simulink model "hybrid_gwo_pso_mppt_grid_det"  (R2024a)
settings: Solver=FixedStepDiscrete  StartTime=0.0  StopTime=2.5  RelTol=1e-3
PreLoadFcn:
  | Ts_Power=1e-6;
  | Ts_Control=100e-6;
undefined symbols (not defined in the file or in its folder): D1, Delta, sigbuilder_block
libraries: spsSeriesRLCBranchLib x5, spsMeanLib x3, spsThreePhaseTransformerTwoWindingsLib x2, spsDistributedParametersLineLib x2, spsThreePhaseParallelRLCLoadLib x2, slpidlib x2, spsabctodq0Lib x2, spsVoltageMeasurementLib x2, spsPWMGeneratorDCDCLib x1, spsThreePhaseSeriesRLCLoadLib x1, spsThreeLevelBridgeLib x1, spsThreePhaseSourceLib x1
(part 2 of 2)

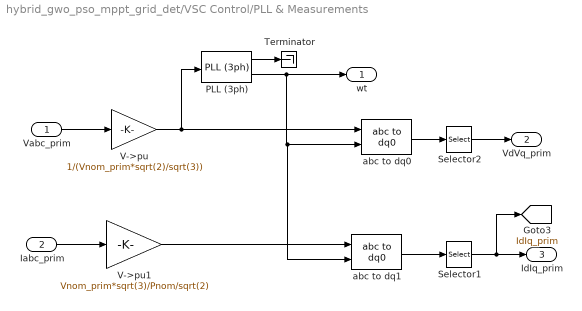
== system hybrid_gwo_pso_mppt_grid_det/VSC Control/PLL & Measurements ==
  Vabc_prim : Inport
  Iabc_prim : Inport  Port=2
  PLL (3ph) : spsPLL3phLib/PLL (3ph)  Fmin=45  Par_Init="[-0.57  Fnom]"  ParK=[180, 3200, 1]  TcD=1e-4  MaxRateChangeFreq=12  FilterCutOffFreq=25  Ts=Ts  AGC=on
  Selector1 : Selector  InputPortWidth=3  IndexOptions=Index vector (dialog)  Indices=[1 2]  OutputSizes=1
  Selector2 : Selector  InputPortWidth=3  IndexOptions=Index vector (dialog)  Indices=[1 2]  OutputSizes=1
  Terminator : Terminator
  V->pu : Gain  Gain=1/(Vnom_prim*sqrt(2)/sqrt(3))  SaturateOnIntegerOverflow=on  OutDataTypeStr=Inherit: Same as input  ParamDataTypeStr=Inherit: Same as input
  V->pu1 : Gain  Gain=Vnom_prim*sqrt(3)/Pnom/sqrt(2)  SaturateOnIntegerOverflow=on  OutDataTypeStr=Inherit: Same as input  ParamDataTypeStr=Inherit: Same as input
  abc to dq0 : spsabctodq0Lib/abc to dq0  Alignment=90 degrees behind phase A axis
  abc to dq1 : spsabctodq0Lib/abc to dq0  Alignment=90 degrees behind phase A axis
  wt : Outport  VectorParamsAs1DForOutWhenUnconnected=off
  VdVq_prim : Outport  Port=2  VectorParamsAs1DForOutWhenUnconnected=off
  IdIq_prim : Outport  Port=3  VectorParamsAs1DForOutWhenUnconnected=off
  tag scope: IdIq_prim=global
  wires:
  V->pu1/1 -> abc to dq1/1
  V->pu/1 -> PLL (3ph)/1, abc to dq0/1
  abc to dq1/1 -> Selector1/1
  Vabc_prim/1 -> V->pu/1
  Iabc_prim/1 -> V->pu1/1
  abc to dq0/1 -> Selector2/1
  Selector2/1 -> VdVq_prim/1
  Selector1/1 -> [IdIq_prim], IdIq_prim/1
  PLL (3ph)/2 -> wt/1, abc to dq1/2, abc to dq0/2
  PLL (3ph)/1 -> Terminator/1

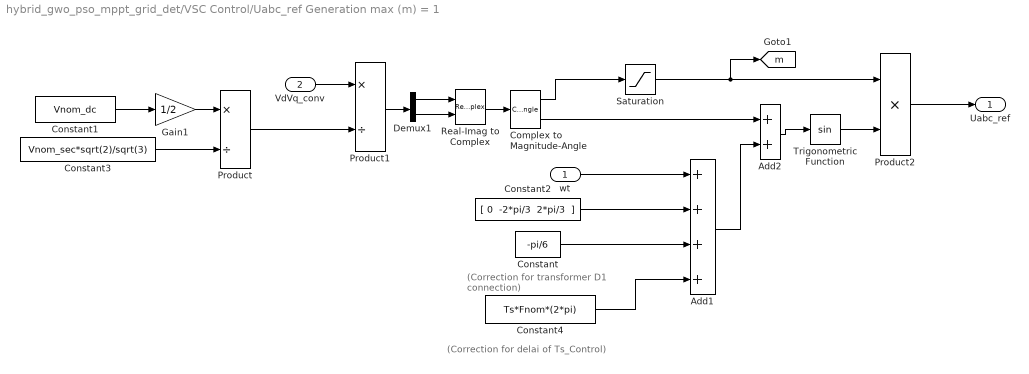
== system hybrid_gwo_pso_mppt_grid_det/VSC Control/Uabc_ref Generation max (m) = 1 ==
  note: (Correction for transformer
      |  D1 connection)
  note: (Correction for delai of Ts_Control)
  wt : Inport
  VdVq_conv : Inport  Port=2
  Add1 : Sum  Inputs=++++
  Add2 : Sum
  Complex to Magnitude-Angle : ComplexToMagnitudeAngle
  Constant : Constant  Value=-pi/6
  Constant1 : Constant  Value=Vnom_dc
  Constant2 : Constant  Value="[ 0  -2*pi/3  2*pi/3  ]"
  Constant3 : Constant  Value=Vnom_sec*sqrt(2)/sqrt(3)
  Constant4 : Constant  Value=Ts*Fnom*(2*pi)
  Demux1 : Demux  Outputs=2
  Gain1 : Gain  Gain=1/2
  Product : Product  Inputs=*/  RndMeth=Zero
  Product1 : Product  Inputs=*/  RndMeth=Zero
  Product2 : Product  Inputs=**  RndMeth=Zero
  Real-Imag to Complex : RealImagToComplex
  Saturation : Saturate  UpperLimit=1  LowerLimit=0
  Trigonometric Function : Trigonometry
  Uabc_ref : Outport  VectorParamsAs1DForOutWhenUnconnected=off
  tag scope: m=global
  wires:
  Complex to Magnitude-Angle/1 -> Saturation/1
  Constant1/1 -> Gain1/1
  VdVq_conv/1 -> Product1/1
  Product1/1 -> Demux1/1
  Gain1/1 -> Product/1
  Real-Imag to Complex/1 -> Complex to Magnitude-Angle/1
  Demux1/1 -> Real-Imag to Complex/1
  Demux1/2 -> Real-Imag to Complex/2
  Constant2/1 -> Add1/2
  Constant/1 -> Add1/3
  Constant3/1 -> Product/2
  Product/1 -> Product1/2
  Complex to Magnitude-Angle/2 -> Add2/1
  Add1/1 -> Add2/2
  Add2/1 -> Trigonometric Function/1
  Saturation/1 -> [m], Product2/1
  Trigonometric Function/1 -> Product2/2
  Product2/1 -> Uabc_ref/1
  wt/1 -> Add1/1
  Constant4/1 -> Add1/4

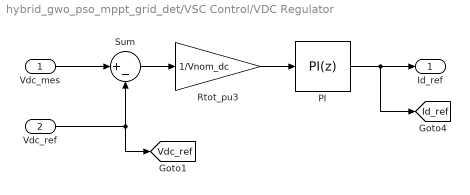
== system hybrid_gwo_pso_mppt_grid_det/VSC Control/VDC Regulator ==
  Vdc_mes : Inport  PortDimensions=1
  Vdc_ref : Inport  Port=2  PortDimensions=1
  PI : slpidlib/PID Controller  Controller=PI  Form=Parallel  TimeDomain=Discrete-time  UseExternalTs=off  SampleTime=Ts  IntegratorMethod=Trapezoidal  FilterMethod=Forward Euler  ControllerParametersSource=internal  P=Kp_VDCreg  I=Ki_VDCreg  UseKiTs=off  D=0  UseExternalDerivativeSource=off  N=100  UseFilter=on  TunerSelectOption=Transfer Function Based (PID Tuner App)  InitialConditionSource=internal  InitialConditionForIntegrator=0  InitialConditionForFilter=0  DifferentiatorICPrevScaledInput=0  ExternalReset=none  TrackingMode=off  Kt=1  LimitOutput=on  SatLimitsSource=internal  UpperSaturationLimit=1.5  LowerSaturationLimit=-1.5  LinearizeAsGain=off  AntiWindupMode=none  Kb=1  LimitIntegrator=off  UpperIntegratorSaturationLimit=inf  LowerIntegratorSaturationLimit=-inf  POutMin=[]  POutMax=[]  IOutMin=[]  IOutMax=[]  DOutMin=[]  DOutMax=[]  NOutMin=[]  NOutMax=[]  SumOutMin=[]  SumOutMax=[]  SaturationOutMin=[]  SaturationOutMax=[]  PParamMin=[]  PParamMax=[]  IParamMin=[]  IParamMax=[]  DParamMin=[]  DParamMax=[]  NParamMin=[]  NParamMax=[]  KbParamMin=[]  KbParamMax=[]  KtParamMin=[]  KtParamMax=[]  KbOutMin=[]  KbOutMax=[]  KtOutMin=[]  KtOutMax=[]  IntegratorOutMin=[]  IntegratorOutMax=[]  FilterOutMin=[]  FilterOutMax=[]  SumI1OutMin=[]  SumI1OutMax=[]  SumI2OutMin=[]  SumI2OutMax=[]  SumI3OutMin=[]  SumI3OutMax=[]  SumI4OutMin=[]  SumI4OutMax=[]  SumDOutMin=[]  SumDOutMax=[]  DifferentiatorOutMin=[]  DifferentiatorOutMax=[]  FilterDiffOutCoefMin=[]  FilterDiffOutCoefMax=[]  ReciprocalOutMin=[]  ReciprocalOutMax=[]  SumDenOutMin=[]  SumDenOutMax=[]  SumNumOutMin=[]  SumNumOutMax=[]  DivideOutMin=[]  DivideOutMax=[]  UdiffTsProdOutMin=[]  UdiffTsProdOutMax=[]  NTsProdOutMin=[]  NTsProdOutMax=[]  UintegralTsProdOutMin=[]  UintegralTsProdOutMax=[]  UngainTsProdOutMin=[]  UngainTsProdOutMax=[]  ClampingZeroOutDataTypeStr=Inherit: Inherit via back propagation  ClampingZeroOutMin=[]  ClampingZeroOutMax=[]  FilterDenConstantOutDataTypeStr=Inherit: Inherit via back propagation  FilterDenConstantOutMin=[]  FilterDenConstantOutMax=[]  PCopyOutDataTypeStr=Inherit: Inherit via back propagation  PCopyOutMin=[]  PCopyOutMax=[]  NCopyOutDataTypeStr=Inherit: Inherit via back propagation  NCopyOutMin=[]  NCopyOutMax=[]  IntegratorContinuousStateAttributes=''  IntegratorStateMustResolveToSignalObject=off  IntegratorRTWStateStorageClass=Auto  FilterContinuousStateAttributes=''  FilterStateMustResolveToSignalObject=off  FilterRTWStateStorageClass=Auto  ParallelPVariant=InternalParameters  IdealPVariant=Disabled  IVariant=InternalParameters  DVariant=Disabled  IntegratorVariant=Discrete  SatVariant=Enabled  AWVariant=Passthrough  PCopyVariant=Disabled  TRVariant=Disabled  FdbkBlocksVariant=Forward  IdealPFdbkVariant=Disabled  SatFdbkVariant=Disabled  DerivativeFilterVariant=Disabled  NVariant=Disabled  NCopyVariant=Disabled_SignalSpec  FilterICVariant=Disabled  IntegratorICVariant=InternalICs  ExternalResetVariant=Disabled  TRSumVariant=Passthrough  SumFdbkVariant=Disabled  SumVariant=Sum_PI  TsampFilterVariant=InternalTs  TsampNgainVariant=Passthrough  TsampIntegralVariant=Disabled_SignalSpec  ExternalSaturationOutDataTypeStr=Inherit: Same as second input  DerivativeSourceVariant=Disabled
  Rtot_pu3 : Gain  Gain=1/Vnom_dc  SaturateOnIntegerOverflow=on  OutDataTypeStr=Inherit: Same as input  ParamDataTypeStr=Inherit: Same as input
  Sum : Sum  Inputs=|+-
  Id_ref : Outport  SampleTime=Ts  InitialOutput=0  VectorParamsAs1DForOutWhenUnconnected=off
  tag scope: Id_ref=global, Vdc_ref=global
  wires:
  Sum/1 -> Rtot_pu3/1
  Vdc_mes/1 -> Sum/1
  Vdc_ref/1 -> Sum/2, [Vdc_ref]
  Rtot_pu3/1 -> PI/1
  PI/1 -> [Id_ref], Id_ref/1

== matlab function hybrid_gwo_pso_mppt_grid_det/ MPPT Controller using GWOPSO /MPPT/MPPT Controller using GWOPSO  ==
  settings: updateMethod=DISCRETE  sampleTime=Ts_Control
  data: Vpv input; Ipv input; Enabled input; D output
%%
% * Author:  Eng. Salah Abbas Taha (S.A.Taha)(salahabbas041@gmail,com,07748191514,Tele.@Eng_441)
% * Date: 06.11.2024
function D = Hybrid_GWO_PSO(Vpv, Ipv,Enabled)
Dinit = 0.5;
SearchAgents_no=6;   % Number of search agents
Max_iteration=10;    % Maximum numbef of iterations
lb = 0.3;            % lb is the lower bound: lb=[lb_1,lb_2,...,lb_d]
ub = 0.9;            % up is the uppper bound: ub=[ub_1,ub_2,...,ub_d]
w=0.5;
a=2;
power_delta =0.01;


% initialize alpha, beta, and delta_pos
persistent params;

if isempty(params)
    params = initialize(SearchAgents_no,lb,ub); 
end



    
% Calculate power
fitness = Vpv * Ipv; 

% Weather conditions test 
if params.runing==false
    
    if abs(fitness - params.power_last) / params.power_last >= power_delta
        params = initialize(SearchAgents_no,lb,ub); 
    else
        D = params.Alpha_pos;
        params.power_last = fitness;
        return;
    end
        
end

params.power_last = fitness;
params.fitness(params.index) = fitness; % Store fitness for the current wolf

% Output duty cycle for the current wolf
D = params.Positions(params.index);

% Step 2: Check if all wolves have been evaluated
params.index = params.index + 1;



if params.index > SearchAgents_no
    
    % Reset index after evaluating all wolves
    params.index = 1; 
    params.iter = params.iter + 1;
    
    % Update dominant levels (alpha, beta, delta)
    [sorted_fitness, sorted_idx] = sort(params.fitness, 'descend');
    params.Alpha_score = sorted_fitness(1); 
    params.Alpha_pos = params.Positions(sorted_idx(1));
    params.Beta_score = sorted_fitness(2); 
    params.Beta_pos = params.Positions(sorted_idx(2));
    params.Delta_score = sorted_fitness(3); 
    params.Delta_pos = params.Positions(sorted_idx(3));
    
    
   
    
    
    for i=1:size(params.Positions,1)
        
        r1=rand(); % r1 is a random number in [0,1]
        r2=rand(); % r2 is a random number in [0,1]
        r3=rand(); % r3 is a random number in [0,1]
        
        A1=2*a*r1-a; 
        C1=2*r2; 
        D_alpha=abs(C1*params.Alpha_pos-w*params.Positions(i)); 
        X1=params.Alpha_pos-A1*D_alpha; 

  
        A2=2*a*r1-a; 
        C2=2*r2; 
        D_beta=abs(C2*params.Beta_pos-w*params.Positions(i)); 
        X2=params.Beta_pos-A2*D_beta; 

       
        A3=2*a*r1-a; 
        C3=2*r2;
        D_delta=abs(C3*params.Delta_pos-w*params.Positions(i)); 
        X3=params.Delta_pos-A3*D_delta; 

        % velocity updation
        params.velocity(i)=w*(params.velocity(i)+C1*r1*(X1-params.Positions(i))+C2*r2*(X2-params.Positions(i))+C3*r3*(X3-params.Positions(i)));
        % positions update
        newPosition = params.Positions(i)+params.velocity(i);
        
        % Enforce boundaries on duty cycle
        if newPosition > ub
            newPosition = ub;
        elseif newPosition < lb
            newPosition = lb;
        end
        
        params.Positions(i)=newPosition;
                   
    end%end for.
    
    
    % Check termination conditions
    if params.iter >= Max_iteration 
%         fprintf('Converged or Max Iterations Reached\n');
        params.runing = false;
        D = params.Alpha_pos;
    end
 
    
end%end if.

if Enabled==0
    D = Dinit;
end


end%end function.


function params = initialize(SearchAgents_no,lb,ub)

params.Alpha_pos= 0;
params.Alpha_score = 0; 

params.Beta_pos=0;
params.Beta_score=0; 
params.Delta_pos=0;
params.Delta_score=0;

%Initialize the positions of search agents
params.Positions= rand(SearchAgents_no,1).*(ub-lb)+lb;
params.fitness = zeros(1,SearchAgents_no); % Fitness values (power values)
params.velocity = zeros(SearchAgents_no,1) ;%0.3*randn(SearchAgents_no,1) ;
params.iter=0;
params.index = 1;
params.runing = true;
params.power_last =0;

end%end function.
